simulink model "gm_majorChangeShift"  (R2022a)
settings: Solver=VariableStepAuto  StartTime=0.0  StopTime=18  RelTol=1e-3
PostLoadFcn:
  | postLoadCallback
InitFcn:
  | initCallback
StopFcn:
  | stopCallback
undefined symbols (not defined in the file or in its folder): modelParams
libraries: dspsigops x15, embmathops x4, hdlsllib x4, dspsrcs4 x3, hdlmdlgenlib x1
settings Model: SimulationMode=accelerator  Creator=Ronnel  LastModifiedBy=Ronnel
settings DataIOCC: ReturnWorkspaceOutputs=off
settings OptimizationCC: BlockReduction=off  ConditionallyExecuteInputs=off  DefaultParameterBehavior=Inlined
settings DebuggingCC: AlgebraicLoopMsg=error  InheritedTsInSrcMsg=none
settings HardwareCC: ProdBitPerPointer=32  ProdBitPerSizeT=32  ProdBitPerPtrDiffT=32  ProdLargestAtomicFloat=None  ProdIntDivRoundTo=Undefined  ProdEndianess=Unspecified  ProdWordSize=32  ProdHWDeviceType=ASIC/FPGA->ASIC/FPGA  TargetBitPerPointer=64  TargetBitPerSizeT=64  TargetBitPerPtrDiffT=64  TargetLongLongMode=on  TargetIntDivRoundTo=Zero  TargetEndianess=LittleEndian  TargetWordSize=64  TargetHWDeviceType=Custom Processor->MATLAB Host Computer  ProdEqTarget=off

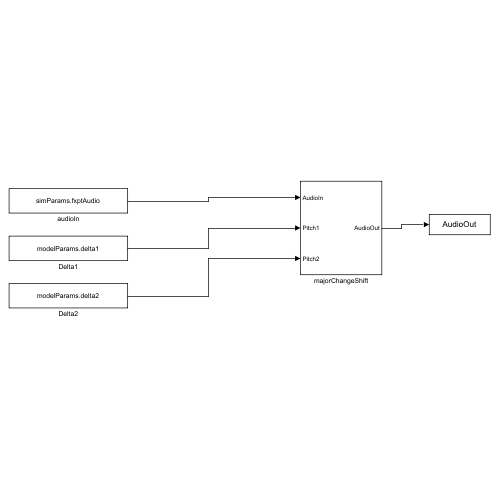
[thumbnail: Simulink's stored preview of the top-level diagram]
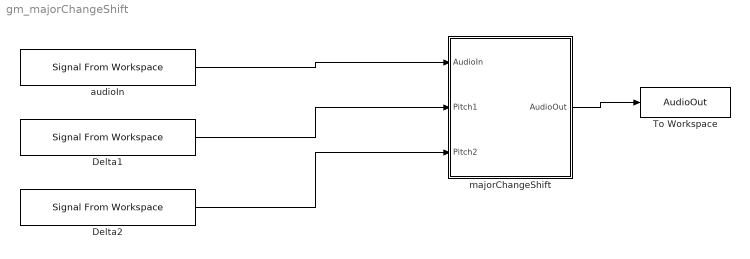
== system gm_majorChangeShift ==
  Delta1 : dspsrcs4/Signal From Workspace  X=modelParams.delta1  Ts=modelParams.audio.samplePeriod  nsamps=1  OutputAfterFinalValue=Holding final value  ignoreOrWarnInputAndFrameLengths=off  OutputFrames=off
  Delta2 : dspsrcs4/Signal From Workspace  X=modelParams.delta2  Ts=modelParams.audio.samplePeriod  nsamps=1  OutputAfterFinalValue=Holding final value  ignoreOrWarnInputAndFrameLengths=off  OutputFrames=off
  To Workspace : ToWorkspace  VariableName=AudioOut  SampleTime=modelParams.audio.samplePeriod
      settings: Save2DSignal=2-D array (concatenate along first dimension)
  audioIn : dspsrcs4/Signal From Workspace  X=simParams.fxptAudio  Ts=modelParams.audio.samplePeriod  nsamps=1  OutputAfterFinalValue=Holding final value  ignoreOrWarnInputAndFrameLengths=off  OutputFrames=off
  majorChangeShift : Subsystem
  wires:
  Delta2/1 -> majorChangeShift/3(Pitch2)
  Delta1/1 -> majorChangeShift/2(Pitch1)
  majorChangeShift/1(AudioOut) -> To Workspace/1
  audioIn/1 -> majorChangeShift/1(AudioIn)

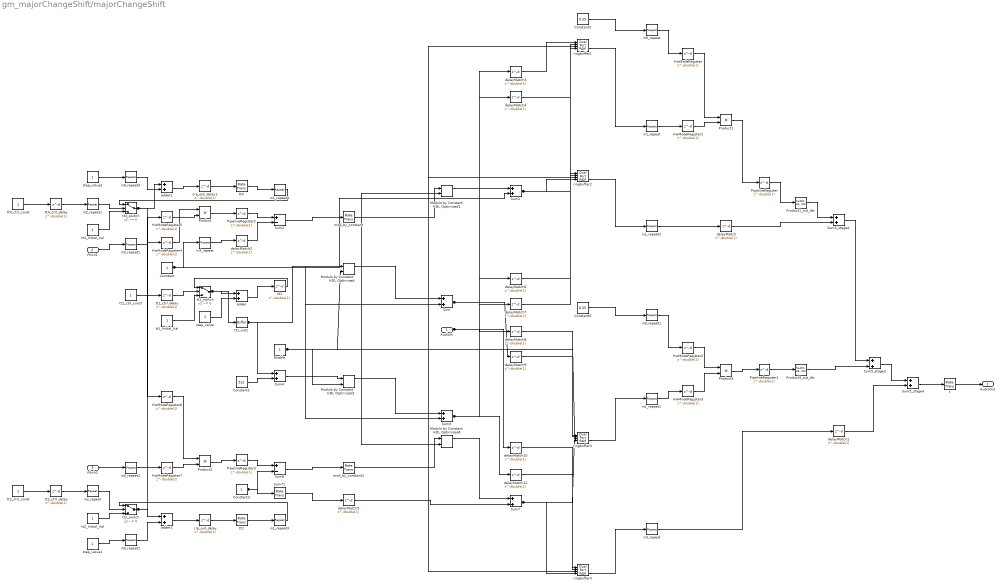
== system gm_majorChangeShift/majorChangeShift ==
  AudioIn : Inport  OutDataTypeStr=fixdt(1, 24, 23)  PortDimensions=1  SampleTime=2.08333333333333e-05
  Pitch1 : Inport  Port=2  OutDataTypeStr=fixdt(1, 24, 23)  PortDimensions=1  SampleTime=2.08333333333333e-05
  Pitch2 : Inport  Port=3  OutDataTypeStr=fixdt(1, 24, 23)  PortDimensions=1  SampleTime=2.08333333333333e-05
  Constant : Constant  OutDataTypeStr=uint32  SampleTime=2.08333333333333e-05
  Constant1 : Constant  Value=512  OutDataTypeStr=uint32  SampleTime=2.08333333333333e-05
  Constant2 : Constant  Value=0.25  OutDataTypeStr=fixdt(0, 24, 23)  SampleTime=2.08333333333333e-05
  Constant3 : Constant  OutDataTypeStr=uint32  SampleTime=1.01725260416667e-08
  Constant5 : Constant  Value=0.25  OutDataTypeStr=fixdt(0, 24, 23)  SampleTime=2.08333333333333e-05
  Enable : Constant  OutDataTypeStr=boolean  SampleTime=2.08333333333333e-05
  HwModeRegister{,1..7} (8 alike) : Delay  DelayLength=double(1)  InitialCondition=0  SampleTime=1.01725260416667e-08
  Modulo by Constant HDL Optimized{,1..2,4} (4 alike) : embmathops/Modulo by Constant HDL Optimized  Denominator=modelParams.buffer_size  SimulateUsing=Code generation
      settings: SourceProductBaseCode=SL
  PipelineRegister{,1..3} (4 alike) : Delay  DelayLength=double(1)  InitialCondition=0  SampleTime=1.01725260416667e-08
  Product : Product  Inputs=**  OutDataTypeStr=fixdt(1, 56, 23)  SampleTime=1.01725260416667e-08
  Product1 : Product  Inputs=**  OutDataTypeStr=fixdt(1, 48, 46)  SampleTime=1.01725260416667e-08
  Product1_out_dtc : DataTypeConversion  OutDataTypeStr=fixdt(1, 24, 23)  SampleTime=1.01725260416667e-08  RndMeth=Floor
  Product2 : Product  Inputs=**  OutDataTypeStr=fixdt(1, 56, 23)  SampleTime=1.01725260416667e-08
  Product3 : Product  Inputs=**  OutDataTypeStr=fixdt(1, 48, 46)  SampleTime=1.01725260416667e-08
  Product3_out_dtc : DataTypeConversion  OutDataTypeStr=fixdt(1, 24, 23)  SampleTime=1.01725260416667e-08  RndMeth=Floor
  Sum{,1,3..4,7} (5 alike) : Sum  AccumDataTypeStr=fixdt(0, 33, 0)  OutDataTypeStr=fixdt(0, 10, 0)  SampleTime=2.08333333333333e-05
  Sum2 : Sum  Inputs=+-  AccumDataTypeStr=fixdt(1, 57, 23)  OutDataTypeStr=fixdt(0, 10, 0)  SampleTime=1.01725260416667e-08
  Sum5_stage2 : Sum  AccumDataTypeStr=fixdt(1, 26, 23)  OutDataTypeStr=fixdt(1, 25, 23)  SaturateOnIntegerOverflow=on  SampleTime=1.01725260416667e-08
  Sum5_stage3 : Sum  AccumDataTypeStr=fixdt(1, 26, 23)  OutDataTypeStr=fixdt(1, 26, 23)  SaturateOnIntegerOverflow=on  SampleTime=1.01725260416667e-08
  Sum5_stage4 : Sum  AccumDataTypeStr=fixdt(1, 26, 23)  OutDataTypeStr=fixdt(1, 24, 23)  SaturateOnIntegerOverflow=on  SampleTime=1.01725260416667e-08
  Sum71 : RateTransition  OutPortSampleTimeOpt=Multiple of input port sample time  OutPortSampleTimeMultiple=2048
  Sum8 : Sum  Inputs=+-  AccumDataTypeStr=fixdt(1, 57, 23)  OutDataTypeStr=fixdt(0, 10, 0)  SampleTime=1.01725260416667e-08
  adder : Sum  AccumDataTypeStr=fixdt(0, 10, 0)  OutDataTypeStr=fixdt(0, 10, 0)  SampleTime=2.08333333333333e-05
  adder1 : Sum  AccumDataTypeStr=uint32  OutDataTypeStr=uint32  SampleTime=1.01725260416667e-08
  adder2 : Sum  AccumDataTypeStr=uint32  OutDataTypeStr=uint32  SampleTime=1.01725260416667e-08
  crp_out_delay : Delay  DelayLength=double(1)  InitialCondition=0  SampleTime=1.01725260416667e-08
  crp_out_delay1 : Delay  DelayLength=double(1)  InitialCondition=0  SampleTime=1.01725260416667e-08
  delayMatch : Delay  DelayLength=double(1)  InitialCondition=0  SampleTime=1.01725260416667e-08
  delayMatch1 : Delay  DelayLength=double(1)  InitialCondition=0  SampleTime=1.01725260416667e-08
  delayMatch{3..11} (9 alike) : Delay  DelayLength=double(1)  InitialCondition=0  SampleTime=2.08333333333333e-05
  delayMatch2 : Delay  DelayLength=double(1)  InitialCondition=0  SampleTime=1.01725260416667e-08
  in0_repeat{,1..3} (4 alike) : dspsigops/Repeat  N=double(2048)  RateOptions=Allow multirate processing  ic=0  mode=Unused parameter value
  in1_repeat{,1..4} (5 alike) : dspsigops/Repeat  N=double(2048)  RateOptions=Allow multirate processing  ic=0  mode=Unused parameter value
  in2_repeat : dspsigops/Repeat  N=double(2048)  RateOptions=Allow multirate processing  ic=0  mode=Unused parameter value
  in2_repeat1 : dspsigops/Repeat  N=double(2048)  RateOptions=Allow multirate processing  ic=0  mode=Unused parameter value
  in3_repeat : dspsigops/Repeat  N=double(2048)  RateOptions=Allow multirate processing  ic=0  mode=Unused parameter value
  in3_repeat1 : dspsigops/Repeat  N=double(2048)  RateOptions=Allow multirate processing  ic=0  mode=Unused parameter value
  in3_repeat2 : dspsigops/Repeat  N=double(2048)  RateOptions=Allow multirate processing  ic=0  mode=Unused parameter value
  in4_repeat : dspsigops/Repeat  N=double(2048)  RateOptions=Allow multirate processing  ic=0  mode=Unused parameter value
  mod_by_constant : RateTransition  OutPortSampleTimeOpt=Multiple of input port sample time  OutPortSampleTimeMultiple=2048
  mod_by_constant1 : RateTransition  OutPortSampleTimeOpt=Multiple of input port sample time  OutPortSampleTimeMultiple=2048
  ringbuffer{1..4} (4 alike) : hdlsllib/HDL RAMs/Dual Port RAM  ram_size=modelParams.dpramAddressSize
      settings: SourceProductBaseCode=SL
  step_value : Constant  VectorParams1D=off  OutDataTypeStr=fixdt(0, 10, 0)  SampleTime=2.08333333333333e-05
  step_value1 : Constant  VectorParams1D=off  OutDataTypeStr=uint32  SampleTime=2.08333333333333e-05
  step_value2 : Constant  VectorParams1D=off  OutDataTypeStr=uint32  SampleTime=2.08333333333333e-05
  t : RateTransition  OutPortSampleTimeOpt=Multiple of input port sample time  OutPortSampleTimeMultiple=2048
  tt1 : Delay  DelayLength=double(1)  InitialCondition=0  SampleTime=2.08333333333333e-05
  tt1_Initial_Val : Constant  OutDataTypeStr=fixdt(0, 10, 0)  SampleTime=2.08333333333333e-05
  tt1_ctrl_const : Constant  OutDataTypeStr=boolean  SampleTime=2.08333333333333e-05
  tt1_ctrl_delay : Delay  DelayLength=double(1)  InitialCondition=0  SampleTime=2.08333333333333e-05
  tt1_out1 : hdlmdlgenlib/Buffer
      settings: SourceProductBaseCode=SL
  tt1_switch : Switch  Criteria=u2 ~= 0  Threshold=double(0)  OutDataTypeStr=fixdt(0, 10, 0)  SampleTime=2.08333333333333e-05  SaturateOnIntegerOverflow=off  InputSameDT=off
  tt2 : RateTransition  OutPortSampleTimeOpt=Multiple of input port sample time  OutPortSampleTimeMultiple=2048
  tt2_Initial_Val : Constant  OutDataTypeStr=uint32  SampleTime=1.01725260416667e-08
  tt2_ctrl_const : Constant  OutDataTypeStr=boolean  SampleTime=2.08333333333333e-05
  tt2_ctrl_delay : Delay  DelayLength=double(1)  InitialCondition=0  SampleTime=2.08333333333333e-05
  tt2_switch : Switch  Criteria=u2 ~= 0  Threshold=double(0)  OutDataTypeStr=uint32  SampleTime=1.01725260416667e-08  SaturateOnIntegerOverflow=off  InputSameDT=off
  tt4 : RateTransition  OutPortSampleTimeOpt=Multiple of input port sample time  OutPortSampleTimeMultiple=2048
  tt4_Initial_Val : Constant  OutDataTypeStr=uint32  SampleTime=1.01725260416667e-08
  tt4_ctrl_const : Constant  OutDataTypeStr=boolean  SampleTime=2.08333333333333e-05
  tt4_ctrl_delay : Delay  DelayLength=double(1)  InitialCondition=0  SampleTime=2.08333333333333e-05
  tt4_switch : Switch  Criteria=u2 ~= 0  Threshold=double(0)  OutDataTypeStr=uint32  SampleTime=1.01725260416667e-08  SaturateOnIntegerOverflow=off  InputSameDT=off
  AudioOut : Outport  SampleTime=2.08333333333333e-05
  wires:
  delayMatch3/1 -> ringbuffer1/1
  Pitch1/1 -> in3_repeat1/1
  Pitch2/1 -> in3_repeat2/1
  Modulo by Constant HDL Optimized/1 -> Sum/1
  Modulo by Constant HDL Optimized1/1 -> Sum1/1
  Modulo by Constant HDL Optimized2/1 -> Sum3/1
  Modulo by Constant HDL Optimized4/1 -> Sum7/1
  ringbuffer1/2 -> in1_repeat/1
  ringbuffer2/2 -> in1_repeat2/1
  ringbuffer3/2 -> in1_repeat1/1
  ringbuffer4/2 -> in3_repeat/1
  step_value1/1 -> in0_repeat2/1
  Constant5/1 -> in0_repeat1/1
  Constant2/1 -> in0_repeat/1
  delayMatch5/1 -> Sum7/2
  step_value2/1 -> in0_repeat3/1
  step_value/1 -> adder/2
  Constant/1 -> Sum3/2, Sum/2, Sum1/2, in4_repeat/1
  tt1_ctrl_delay/1 -> tt1_switch/2
  tt2_ctrl_delay/1 -> in2_repeat/1
  tt4_ctrl_delay/1 -> in2_repeat1/1
  tt1_ctrl_const/1 -> tt1_ctrl_delay/1
  tt1_Initial_Val/1 -> tt1_switch/3
  tt1_switch/1 -> tt1_out1/1, adder/1
  tt1_out1/1 -> Sum4/1, Modulo by Constant HDL Optimized/1
  Constant1/1 -> Sum4/2
  Sum4/1 -> Modulo by Constant HDL Optimized2/1
  Enable/1 -> Modulo by Constant HDL Optimized/2, Modulo by Constant HDL Optimized1/2, Modulo by Constant HDL Optimized2/2, Modulo by Constant HDL Optimized4/2, ringbuffer1/3, ringbuffer2/3, ringbuffer3/3, ringbuffer4/3
  delayMatch4/1 -> ringbuffer1/2
  delayMatch7/1 -> ringbuffer2/2
  tt2_ctrl_const/1 -> tt2_ctrl_delay/1
  Sum1/1 -> ringbuffer1/4, ringbuffer2/4
  tt4_ctrl_const/1 -> tt4_ctrl_delay/1
  Sum7/1 -> ringbuffer3/4, ringbuffer4/4
  mod_by_constant/1 -> Modulo by Constant HDL Optimized1/1
  Product1_out_dtc/1 -> Sum5_stage2/1
  mod_by_constant1/1 -> Modulo by Constant HDL Optimized4/1
  Product3_out_dtc/1 -> Sum5_stage3/2
  t/1 -> AudioOut/1
  delayMatch6/1 -> ringbuffer2/1
  delayMatch9/1 -> ringbuffer3/2
  Sum71/1 -> delayMatch5/1
  delayMatch8/1 -> ringbuffer3/1
  delayMatch11/1 -> ringbuffer4/2
  delayMatch10/1 -> ringbuffer4/1
  Sum/1 -> delayMatch9/1, delayMatch4/1
  AudioIn/1 -> delayMatch10/1, delayMatch8/1, delayMatch6/1, delayMatch3/1
  Sum3/1 -> delayMatch11/1, delayMatch7/1
  adder/1 -> tt1/1
  tt1/1 -> tt1_switch/1
  tt2/1 -> in1_repeat3/1
  tt4/1 -> in1_repeat4/1
  in0_repeat/1 -> HwModeRegister/1
  in1_repeat/1 -> HwModeRegister1/1
  PipelineRegister/1 -> Product1_out_dtc/1
  in0_repeat1/1 -> HwModeRegister2/1
  in1_repeat1/1 -> HwModeRegister3/1
  PipelineRegister1/1 -> Product3_out_dtc/1
  in1_repeat2/1 -> delayMatch/1
  in3_repeat/1 -> delayMatch1/1
  Sum5_stage4/1 -> t/1
  delayMatch/1 -> Sum5_stage2/2
  delayMatch1/1 -> Sum5_stage4/2
  Sum5_stage2/1 -> Sum5_stage3/1
  Sum5_stage3/1 -> Sum5_stage4/1
  in0_repeat2/1 -> adder1/2
  in1_repeat3/1 -> tt2_switch/1
  in2_repeat/1 -> tt2_switch/2
  in3_repeat1/1 -> HwModeRegister5/1
  in4_repeat/1 -> delayMatch2/1
  crp_out_delay/1 -> tt2/1
  Sum2/1 -> mod_by_constant/1
  tt2_Initial_Val/1 -> tt2_switch/3
  adder1/1 -> crp_out_delay/1
  tt2_switch/1 -> adder1/1, HwModeRegister4/1
  PipelineRegister2/1 -> Sum2/1
  delayMatch2/1 -> Sum2/2
  in0_repeat3/1 -> adder2/2
  in1_repeat4/1 -> tt4_switch/1
  in2_repeat1/1 -> tt4_switch/2
  in3_repeat2/1 -> HwModeRegister7/1
  crp_out_delay1/1 -> tt4/1
  Constant3/1 -> Sum71/1, Sum8/2
  Sum8/1 -> mod_by_constant1/1
  tt4_Initial_Val/1 -> tt4_switch/3
  adder2/1 -> crp_out_delay1/1
  tt4_switch/1 -> adder2/1, HwModeRegister6/1
  PipelineRegister3/1 -> Sum8/1
  Product1/1 -> PipelineRegister/1
  HwModeRegister/1 -> Product1/1
  HwModeRegister1/1 -> Product1/2
  Product3/1 -> PipelineRegister1/1
  HwModeRegister2/1 -> Product3/1
  HwModeRegister3/1 -> Product3/2
  Product/1 -> PipelineRegister2/1
  HwModeRegister4/1 -> Product/1
  HwModeRegister5/1 -> Product/2
  Product2/1 -> PipelineRegister3/1
  HwModeRegister6/1 -> Product2/1
  HwModeRegister7/1 -> Product2/2
